simulink model "Ex_3_sim_test"  (R2021a)
settings: Solver=VariableStepAuto  StartTime=0.0  StopTime=200  RelTol=1e-3
settings Model: Creator=david  LastModifiedBy=david

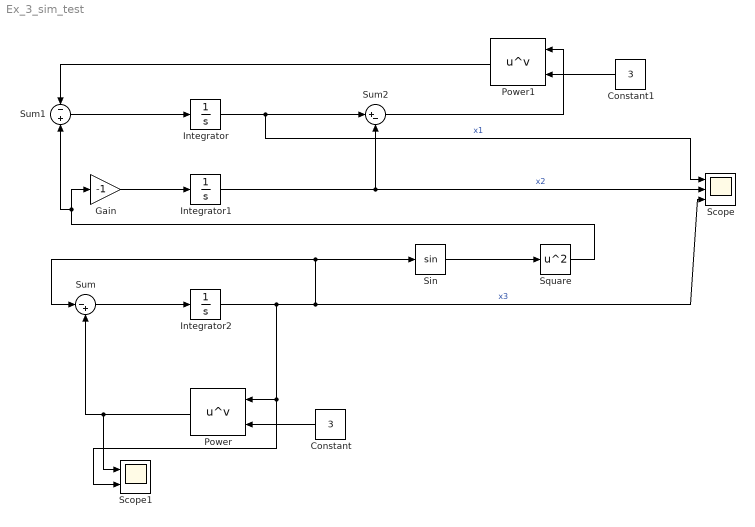
== system Ex_3_sim_test ==
  Constant : Constant  Value=3
  Constant1 : Constant  Value=3
  Gain : Gain  Gain=-1
  Integrator : Integrator  InitialCondition=10
  Integrator1 : Integrator  InitialCondition=-10
  Integrator2 : Integrator  InitialCondition=0.3
  Power : Math  Operator=pow  SaturateOnIntegerOverflow=on
  Power1 : Math  Operator=pow  SaturateOnIntegerOverflow=on
  Scope : Scope  NumInputPorts=3
  Scope1 : Scope  NumInputPorts=2
  Sin : Trigonometry
  Square : Math  Operator=square  SaturateOnIntegerOverflow=on
  Sum : Sum  Inputs=|-+
  Sum1 : Sum  Inputs=-|+
  Sum2 : Sum  Inputs=|+-
  wires:
  Sum1/1 -> Integrator/1
  Integrator/1 -> Scope/1, Sum2/1  "x1"
  Integrator2/1 -> Scope1/2, Power/1, Sum/1, Sin/1, Scope/3  "x3"
  Constant/1 -> Power/2
  Power/1 -> Scope1/1, Sum/2
  Sum/1 -> Integrator2/1
  Sin/1 -> Square/1
  Gain/1 -> Integrator1/1
  Square/1 -> Sum1/2, Gain/1
  Integrator1/1 -> Scope/2, Sum2/2  "x2"
  Constant1/1 -> Power1/2
  Power1/1 -> Sum1/1
  Sum2/1 -> Power1/1
